simulink model "Hardware_Simulation_Position_Control"  (R2023a)
settings: Solver=VariableStepAuto  StartTime=0.0  StopTime=18  RelTol=1e-3
undefined symbols (not defined in the file): Ts
libraries: mbedblockslib x3, stm_qeplib x1
settings Model: Creator=Marco  LastModifiedBy=Marco

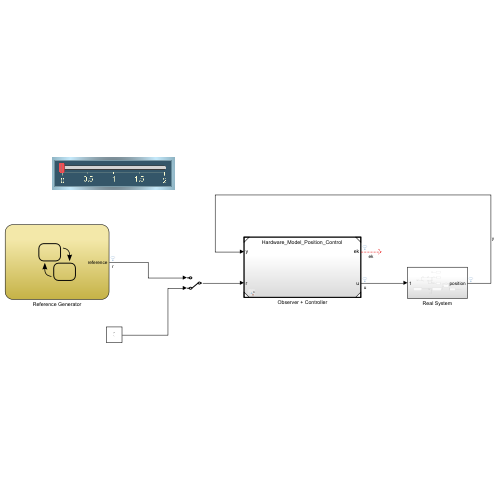
[thumbnail: Simulink's stored preview of the top-level diagram]
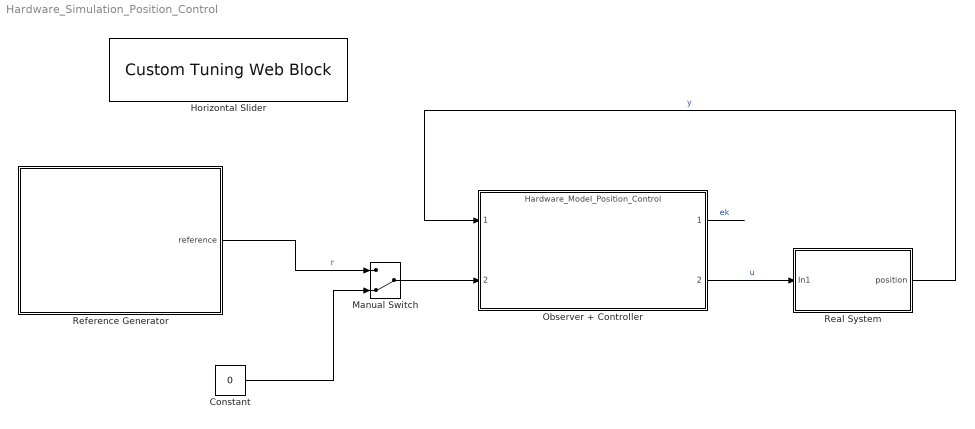
== system Hardware_Simulation_Position_Control ==
  Constant : Constant  Value=0
  Horizontal Slider : CustomTuningWebBlock  LabelPosition=Hide  ShowInitialText=on  Configuration="{\"components\":[{\"name\":\"LinearScaleComponent\",\"settings\":{\"bounds\":{\"max\":2,\"min\":0,\"tickInterval\":\"auto\"},\"internalTickHeightScaleFactor\":0.5,\"labelColor\":[255,255,200],\"labelFont\":{\"font\":\"Arial\",\"fontSize\":12},\"labelOffset\":0.05,\"labelTransparency\":1,\"needleImage\":{\"size\":[596,842],\"src\":\"data:image\\/svg+xml;base64,PD94bWwgdmVyc2lvbj0iMS4wIiBlbmNvZGluZz0idXRmLTgiPz4NCjwhLS0gR2VuZXJhdG9yOiBBZG9iZSBJbGx1c3RyYXRvciAyNS4wLjAsIFNWRyBFeHBvcnQgUGx1Zy1JbiAuIFNWRyBWZXJzaW9uOiA2LjAwIEJ1aWxkIDApICAtLT4NCjxzdmcgdmVyc2lvbj0iMS4xIg0KCSBpZD0ic3ZnOCIgeG1sbnM6Y2M9Imh0dHA6Ly9jcmVhdGl2ZWNvbW1vbnMub3JnL25zIyIgeG1sbnM6ZGM9Imh0dHA6Ly9wdXJsLm9yZy9kYy9lbGVtZW50cy8xLjEvIiB4bWxuczppbmtzY2FwZT0iaHR0cDovL3d3dy5pbmtzY2FwZS5vcmcvbmFtZXNw ...(+2420 chars)\",\"srcOrientation\":\"Right\"},\"needleOffset\":[-0.8044596912521441,-0.0642123287671233],\"needleSize\":{\"height\":0.4337797619047619,\"width\":0.07668067226890757},\"position\":[0.2829861111111111,0.04398634453781513,0.9196428571428571,0.6088789682539683],\"referencePoint\":\"auto\",\"scaleColors\":[],\"scaleColorsSize\":0.2,\"scaleDirection\":\"LR\",\"showLabels\":1,\"showMinorTicks\":0,\"showSpanLine\":1,\"showTicks\":1,\"tickColor\":[252,252,197],\"tickTransparency\":1,\"valueBarColor\":[0,114,189],\"valueBarOffset\":-0.27,\"valueBarSize\":0.1,\"valueBarTransparency\":1}},{\"name\":\"BackgroundImageComponent\",\"settings\":{\"image\":{\"size\":[380,101],\"src\":\"data:image\\/svg+xml;base64,PHN2ZyB4bWxucz0iaHR0cDovL3d3dy53My5vcmcvMjAwMC9zdmciIHhtbG5zOnhsaW5rPSJodHRwOi8vd3d3LnczLm9yZy8xOTk5L3hsaW5rIiB2aWV3Qm94PSIwIDAgMzgwIDEwMSI+PGRlZnM+PHN0eWxlPi5jbHMtMXtmaWxsOiMwMDJiNDI7fS5jbHMtMntmaWxsOiM0MjcwODI7fS5jbHMtM3tmaWxsOnVybCgjcmFkaWFsLWdyYWRpZW50KTt9LmNscy00e2ZpbGw6I2M4YzhjODtzdHJva2U6IzAwMDt9PC9zdHlsZT48cmFkaWFsR3JhZGllbnQgaWQ9InJhZGlhbC1ncmFkaWVudCIgY3g9IjE5MCIgY3k9IjUwLjUiIHI9IjI2OS4yMSIgZ3JhZGllbnRVbml0cz0idXNlclNwYWNlT25Vc2UiPjxzdG9wIG9mZnNldD0iMC4wMSIgc3RvcC1jb2xvcj0iIzNlNGY1OCIvPjxzdG9wIG9mZnNldD0iMC4wNiIgc3RvcC1jb2xvcj0iIzQ0NTc2MSIvPjxzdG9wIG9mZnNldD0iMC4xNSIgc3RvcC1jb2xvcj0iIzU1NmE3NiIvPjxzdG9wIG9mZnNldD0iMC4yNSIgc3RvcC1jb2xvcj0iIzZkODg5NSIvPjxzdG9wIG9mZnNldD0iMC4zOCIgc3RvcC1jb2xvcj0iIzhmYjJjMyIvPjxzdG9wIG9mZnNldD0iMC41MiIgc3RvcC1jb2xvcj0iI2I2ZTRmYSIvPjxzdG9wIG9mZnNldD0iMSIgc3RvcC1jb2xvcj0iIzE1NDY1NyIvPjwvcmFkaWFsR3JhZGllbnQ+PC9kZWZzPjxnIGlkPSJmcmFtZSI+PGcgaWQ9IkxheWVyXzIiIGRhdGEtbmFtZT0iTGF5ZXIgMiI+PGcgaWQ9IkxheWVyXzEtMiIgZGF0YS1uYW1lPSJMYXllciAxLTIiPjxyZWN0IGlkPSJyZWN0MTAzNiIgY2xhc3M9ImNscy0xIiB4PSIxMSIgeT0iMTEiIHdpZHRoPSIzNTgiIGhlaWdodD0iNzkiLz48cGF0aCBpZD0icGF0aDEwMzgiIGNsYXNzPSJjbHMtMiIgZD0iTTgsOFY5M0gzNzJWOFpNMzY5LDkwSDExVjExSDM2OVoiLz48cGF0aCBpZD0icGF0aDEwNDAiIGNsYXNzPSJjbHMtMyIgZD0iTTAsMFYxMDFIMzgwVjBaTTM3Miw5M0g4VjhIMzcyWiIvPjwvZz48L2c+PC9nPjxnIGlkPSJ0cmFjayI+PHBhdGggaWQ9InJlY3QxNjExIiBjbGFzcz0iY2xzLTQiIGQ9Ik0zMy4zNywyNi41OUgzNDYuNjNjNCwwLDcuMjUsMi42LDcuMjUsNS44MWgwYzAsMy4yMS0zLjI1LDUuODItNy4yNSw1LjgySDMzLjM3Yy00LDAtNy4yNS0yLjYxLTcuMjUtNS44MmgwQzI2LjEyLDI5LjE5LDI5LjM3LDI2LjU5LDMzLjM3LDI2LjU5WiIvPjwvZz48L3N2Zz4=\",\"srcOrientation\":\"horizontal\"},\"position\":[0,0,1,1],\"scaleMode\":\"0\"}},{\"name\":\"ForegroundImageComponent\",\"settings\":{\"image\":{\"size\":[0,0],\"src\":\"default\",\"srcOrientation\":[]},\"isForeground\":1,\"position\":[0,0,1,1],\"scaleMode\":\"0\"}}],\"settings\":{\"BindingType\":\"param\",\"aspectRatio\":3.7777777777777777,\"backgroundColor\":[0,0,0,\"1\"],\"backgroundOffset\":0,\"backgroundOpacity\":1,\"fixedAspectRatio\":\"on\",\"foregroundColor\":[252,252,196],\"orientation\":\"horizontal\",\"showBackgroundColor\":false,\"value\":0,\"version\":\"R2023a\"},\"type\":\"LinearGauge\"}"
  Manual Switch : ManualSwitch  CurrentSetting=0
  Observer + Controller : ModelReference  ModelNameDialog=Hardware_Model_Position_Control.slx  SimulationMode=Normal  ModelReferenceVersion=1.15
  Real System : Subsystem
  Reference Generator : Stateflow chart  TreatAsAtomicUnit=on
  wires:
  Real System/1(position) -> Observer + Controller/1  "y"
  Observer + Controller/1 -> ?  "ek"
  Observer + Controller/2 -> Real System/1(In1)  "u"
  Manual Switch/1 -> Observer + Controller/2
  Reference Generator/1(reference) -> Manual Switch/1  "r"
  Constant/1 -> Manual Switch/2

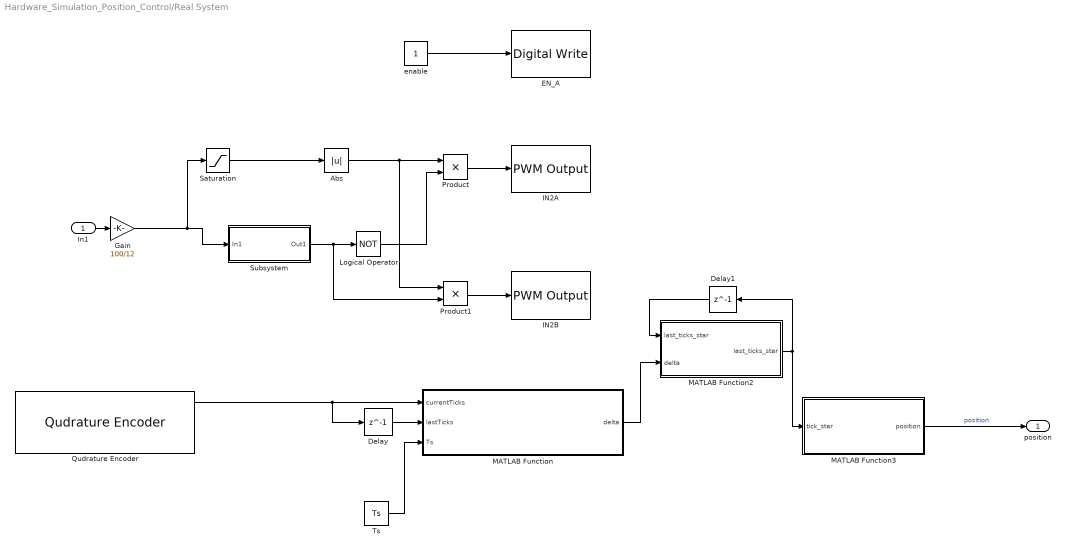
== system Hardware_Simulation_Position_Control/Real System ==
  In1 : Inport
  Abs : Abs  SaturateOnIntegerOverflow=off
  Delay : Delay  DelayLength=1  InitialCondition=0
  Delay1 : Delay  DelayLength=1  InitialCondition=0
  EN_A : mbedblockslib/Digital Write  Pin=2  Direction=output
      settings: LibrarySourceBlock=stmnucleorootlib/Common/Digital Write
  Gain : Gain  Gain=100/12
  IN2A : mbedblockslib/PWM Output  Pin=4  EnableInputFrequency=off  InitialFrequency=PWMFreq  InitialDutyCycle=50  NotificationType=None
      settings: LibrarySourceBlock=stmnucleorootlib/Common/PWM Output
  IN2B : mbedblockslib/PWM Output  Pin=5  EnableInputFrequency=off  InitialFrequency=PWMFreq  InitialDutyCycle=50  NotificationType=None
      settings: LibrarySourceBlock=stmnucleorootlib/Common/PWM Output
  Logical Operator : Logic  Operator=NOT  AllPortsSameDT=off  OutDataTypeStr=boolean
  MATLAB Function : MATLAB Function  TreatAsAtomicUnit=on
  MATLAB Function2 : MATLAB Function  TreatAsAtomicUnit=on
  MATLAB Function3 : MATLAB Function  TreatAsAtomicUnit=on
  Product : Product
  Product1 : Product
  Qudrature Encoder : stm_qeplib/Qudrature Encoder  SampleTime=Ts
  Saturation : Saturate  UpperLimit=100  LowerLimit=-100
  Subsystem : Subsystem
  Ts : Constant  Value=Ts
  enable : Constant
  position : Outport
  wires:
  enable/1 -> EN_A/1
  Subsystem/1(Out1) -> Product1/2, Logical Operator/1
  Saturation/1 -> Abs/1
  Product1/1 -> IN2B/1
  Product/1 -> IN2A/1
  Logical Operator/1 -> Product/2
  Abs/1 -> Product1/1, Product/1
  Gain/1 -> Saturation/1, Subsystem/1(In1)
  MATLAB Function2/1(last_ticks_star) -> MATLAB Function3/1(tick_star), Delay1/1
  Qudrature Encoder/1 -> Delay/1, MATLAB Function/1(currentTicks)
  MATLAB Function/1(delta) -> MATLAB Function2/2(delta)
  Delay1/1 -> MATLAB Function2/1("last_ticks_star ")
  Ts/1 -> MATLAB Function/3(Ts)
  Delay/1 -> MATLAB Function/2(lastTicks)
  In1/1 -> Gain/1
  MATLAB Function3/1(position) -> position/1  "position"

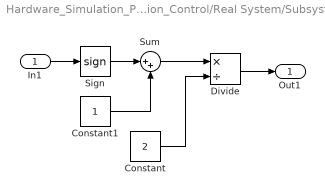
== system Hardware_Simulation_Position_Control/Real System/Subsystem ==
  In1 : Inport
  Constant : Constant  Value=2
  Constant1 : Constant
  Divide : Product  Inputs=*/
  Sign : Signum
  Sum : Sum  Inputs=|++
  Out1 : Outport
  wires:
  In1/1 -> Sign/1
  Sign/1 -> Sum/1
  Constant1/1 -> Sum/2
  Sum/1 -> Divide/1
  Constant/1 -> Divide/2
  Divide/1 -> Out1/1

== stateflow chart Hardware_Simulation_Position_Control/Reference Generator ==
  state Start
    reference = 0;
  state State1
    reference = deg2rad(30)
  state State4
    reference = deg2rad(-30)
  state State2
    reference = deg2rad(180)
  state State3
    reference = deg2rad(-180)
  state State5
    reference = 0
  (default) -> Start
  Start -> State1 : [after(3,sec)]
  State1 -> State4 : [after(3, sec)]
  State4 -> State2 : [after(3,sec)]
  State3 -> Start : [after(3,sec)]
  State2 -> State5 : [after(3,sec)]
  State5 -> State3 : [after(3,sec)]
  data: reference output

== matlab function Hardware_Simulation_Position_Control/Real System/MATLAB Function ==
  data: currentTicks input; delta output; lastTicks input; Ts input
function delta = getTicksDelta(currentTicks, lastTicks, Ts)

currentTicks = double(currentTicks);
lastTicks = double(lastTicks);

if abs(currentTicks - lastTicks) <= ceil(8400*Ts)
    delta = currentTicks-lastTicks;
else
    if lastTicks > currentTicks
        delta = currentTicks + 2^16-1-lastTicks;
    else
        delta = currentTicks - 2^16+1-lastTicks;

end

end

== matlab function Hardware_Simulation_Position_Control/Real System/MATLAB Function2 ==
  data: last_ticks_star input; delta input; last_ticks_star output
function last_ticks_star = modCounter(last_ticks_star,delta)
     sum = last_ticks_star+delta;
	 last_ticks_star = sign(sum)*mod(abs(sum),89796);

end

== matlab function Hardware_Simulation_Position_Control/Real System/MATLAB Function3 ==
  data: tick_star input; position output
function position = getPosition(tick_star)

    ticks_star = double(tick_star);

    position = 2*pi*ticks_star/(3591.84);

end
